simulink model "statikus_linearizalas"  (Simulink 8.7)
settings: Solver=VariableStepAuto  StartTime=0.0  StopTime=t(end)  RelTol=1e-3
values from neighbouring files (symbols this model uses):
  inv_u_stat = y_stat(i-1:end)    [Sebessegszabalyozas_sim.m]
  inv_y_stat = u_stat(i-1:end)    [Sebessegszabalyozas_sim.m]
  K = P1.Kp    [Sebessegszabalyozas_sim.m]
  T = P1.Tp1    [Sebessegszabalyozas_sim.m]
  Ts = 0.01    [Sebessegszabalyozas_sim.m]
  u_sat = y_sat/K    [Sebessegszabalyozas_sim.m]
  u_stat = [0;100;200;250;300;350;400;450;500;550;600;700;750]    [Untitled.m]    (also in ident.mat = [0 100 200 300 400 500 600 700])
  y_stat = y_stat*K    [Sebessegszabalyozas_sim.m]    (also in Untitled.m = [0;  0;  0;  0; 42; 67; 80; 95;110;120;130;160;170]; ident.mat = [0 0 0 32 100 160 216 260])
settings Model: Creator=Mester Ádám  LastModifiedBy=Mester Ádám
settings DataIOCC: LimitDataPoints=off  SaveFormat=Dataset
settings DebuggingCC: UnderspecifiedInitializationDetection=Simplified  MergeDetectMultiDrivingBlocksExec=error
settings HardwareCC: ProdBitPerPointer=64  ProdLargestAtomicFloat=Float  ProdIntDivRoundTo=Zero  ProdEndianess=LittleEndian  ProdWordSize=64  ProdHWDeviceType=Intel->x86-64 (Windows64)
settings ModelReferenceCC: PropagateSignalLabelsOutOfModel=on
settings ConfigComp: CovModelRefEnable=off

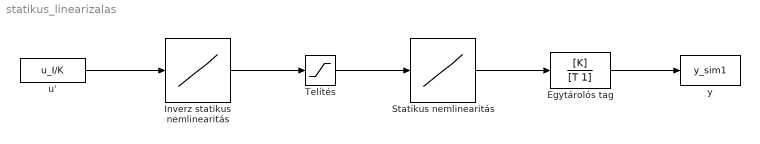
== system statikus_linearizalas ==
  Egytárolós tag : TransferFcn  Numerator=[K]  Denominator=[T 1]
  Inverz statikus nemlinearitás : Lookup_n-D  NumberOfTableDimensions=1  BreakpointsForDimension1=inv_u_stat  Table=inv_y_stat  InternalRulePriority=Speed  RndMeth=Simplest  InputSameDT=on
  Statikus nemlinearitás : Lookup_n-D  NumberOfTableDimensions=1  BreakpointsForDimension1=u_stat  Table=y_stat  InternalRulePriority=Speed  RndMeth=Simplest  InputSameDT=on
  Telítés : Saturate  UpperLimit=u_sat  LowerLimit=0
  u' : FromWorkspace  VariableName=u_I/K  SampleTime=Ts
  y : ToWorkspace  VariableName=y_sim1  SaveFormat=Structure  SampleTime=Ts
  wires:
  Telítés/1 -> Statikus nemlinearitás/1
  Statikus nemlinearitás/1 -> Egytárolós tag/1
  Egytárolós tag/1 -> y/1
  u'/1 -> Inverz statikus nemlinearitás/1
  Inverz statikus nemlinearitás/1 -> Telítés/1
